simulink model "buffal_m"  (Simulink 7.9)
settings: Solver=ode45  SolverMode=SingleTasking  StartTime=0.0  StopTime=999999  MaxStep=10  RelTol=1e-3  AbsTol=1e-3
values from neighbouring files (symbols this model uses):
  U = st_Varia('LongNames')    [buffWQ_i.m]    (also in buffal_i.m; buffer_i.m)
  x0 = zeros(U.Number,1)    [buffWQ_i.m]    (also in buffWQ_s.m = x0; buffal_i.m; buffal_s.m = x0; buffer_s.m = x0)
undefined symbols (not defined in the file or in its folder): B
settings Model: Creator=M.Sparnaaij  LastModifiedBy=M.Sparnaaij
settings DataIOCC: LimitDataPoints=off  SaveOutput=off  SaveTime=off  SignalLoggingName=sigsOut
settings OptimizationCC: BooleanDataType=off
settings DebuggingCC: SaveWithParameterizedLinksMsg=none  SignalResolutionControl=TryResolveAllWithWarning  SolverPrmCheckMsg=none  MultiTaskDSMMsg=warning  MultiTaskCondExecSysMsg=none  StrictBusMsg=None
settings HardwareCC: TargetUnknown=on
settings RTWCC: IncludeERTFirstTime=on
settings GRTTargetCC: CombineOutputUpdateFcns=off  GRTInterface=on

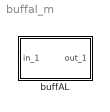
== system buffal_m ==
  buffAL : Subsystem  Description=buffal
      mask init:
      | filenaam='.\StimelaData\buffal_p.mat';
      | 
      | [Pn,Fn,Fext]=Fileprop(filenaam);
      | 
      | errstr = st_UniqName(filenaam,'filenaam=''','SubSystem','OpenFcn');
      | if errstr, error([errstr 'The filename "' filenaam '" is already in use. Choose a different filename.']), end
      | 
      | P = buffal_p(filenaam);
      | [B,x0,U]=buffal_i(filenaam);
      settings: OpenFcn=|
      | filenaam='.\StimelaData\buffal_p.mat';
      | st_ParameterInput('init',gcb,filenaam,'buffal');
      mask Display:
      | plot(0,0,100,100,[0 20],[50 50],[0 20],[55 55],[80 100],[50 50],[80 100],[55 55],[20 80 80 20 20],[10 10 90  90 10]);
      | disp('')
      | text(50,50,'buffal', 'horizontalAlignment', 'center', 'verticalAlignment', 'middle');
      | text(50,0,Fn, 'horizontalAlignment', 'center', 'verticalAlignment', 'base');

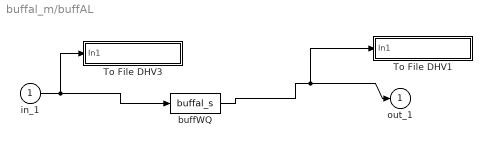
== system buffal_m/buffAL ==
  in_1 : Inport
  To File DHV1 : Subsystem  mask(To File DHV){naam=[filenaam(1:length(filenaam)-4) '_out.sti']}
      mask prompts: naam "Naam van bestand"
      mask init:
      | set_param([gcb '/To File'],'Filename',naam);
      mask Display: disp(naam)
  To File DHV3 : Subsystem  mask(To File DHV){naam=[filenaam(1:length(filenaam)-4) '_in.sti']}
      mask prompts: naam "Naam van bestand"
      mask init:
      | set_param([gcb '/To File'],'Filename',naam);
      mask Display: disp(naam)
  buffWQ : S-Function  FunctionName=buffal_s  Parameters=B,x0,U,P  EnableBusSupport=off
  out_1 : Outport  InitialOutput=0
  wires:
  in_1/1 -> To File DHV3/1(In1), buffWQ/1
  buffWQ/1 -> To File DHV1/1(In1), out_1/1

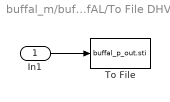
== system buffal_m/buffAL/To File DHV1 ==
  In1 : Inport
  To File : ToFile  Filename=buffal_p_out.sti  MatrixName=buffalout
  wires:
  In1/1 -> To File/1

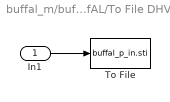
== system buffal_m/buffAL/To File DHV3 ==
  In1 : Inport
  To File : ToFile  Filename=buffal_p_in.sti  MatrixName=buffalin
  wires:
  In1/1 -> To File/1
